simulink model "Galvo_sys_v13"  (R2013a)
settings: Solver=ode45  StartTime=0.0  StopTime=50e-3  MaxStep=1e-4  RelTol=1e-3
InitFcn:
  | Kp_cc = evalin('base','Kp_cc');
StartFcn:
  | Kp_cc = evalin('base','Kp_cc')
model workspace (MATLAB code in the model file):
  | Kp_cc = evalin('base','Kp_cc');
libraries: simulink x2
settings Model: Kp_cc=1  Creator=mainster  LastModifiedBy=mainster
settings DataIOCC: SaveFormat=StructureWithTime

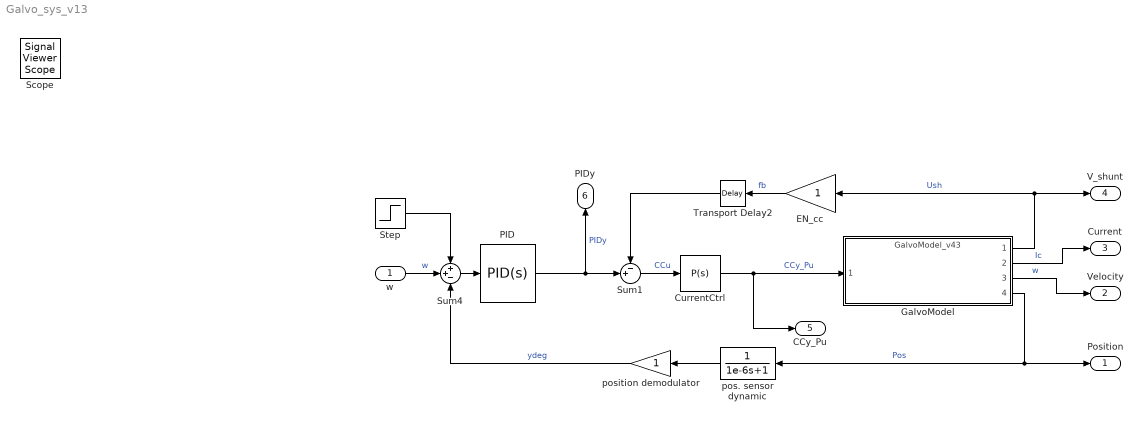
== system Galvo_sys_v13 ==
  w : Inport
  CurrentCtrl : simulink/Continuous/PID Controller  Controller=P  TimeDomain=Continuous-time  SampleTime=1  IntegratorMethod=Forward Euler  FilterMethod=Forward Euler  Form=Parallel  P=Kp_cc  I=1  D=0  N=100  InitialConditionSource=internal  InitialConditionForIntegrator=0  InitialConditionForFilter=0  ExternalReset=none  LimitOutput=on  UpperSaturationLimit=25  LowerSaturationLimit=-25  LinearizeAsGain=on  AntiWindupMode=none  Kb=1  TrackingMode=off  Kt=1  PParamMin=[]  PParamMax=[]  IParamMin=[]  IParamMax=[]  DParamMin=[]  DParamMax=[]  NParamMin=[]  NParamMax=[]  KbParamMin=[]  KbParamMax=[]  KtParamMin=[]  KtParamMax=[]  POutMin=[]  POutMax=[]  IOutMin=[]  IOutMax=[]  DOutMin=[]  DOutMax=[]  NOutMin=[]  NOutMax=[]  KbOutMin=[]  KbOutMax=[]  KtOutMin=[]  KtOutMax=[]  IntegratorOutMin=[]  IntegratorOutMax=[]  FilterOutMin=[]  FilterOutMax=[]  SumOutMin=[]  SumOutMax=[]  SumI1OutMin=[]  SumI1OutMax=[]  SumI2OutMin=[]  SumI2OutMax=[]  SumI3OutMin=[]  SumI3OutMax=[]  SumDOutMin=[]  SumDOutMax=[]  SaturationOutMin=[]  SaturationOutMax=[]  IntegratorContinuousStateAttributes=''  IntegratorStateMustResolveToSignalObject=off  IntegratorRTWStateStorageClass=Auto  FilterContinuousStateAttributes=''  FilterStateMustResolveToSignalObject=off  FilterRTWStateStorageClass=Auto
      settings: AttributesFormatString=Kp_cc = %<P>\nUccLim = +-%<UpperSaturationLimit>
  EN_cc : Gain
  GalvoModel : ModelReference  ModelNameDialog=GalvoModel_v43.slx  SimulationMode=Normal  Variant=on  OverrideUsingVariant=GalvoModel_v43  ModelReferenceVersion=1.40  CopyOfModelName=GalvoModel_v43.slx  DefaultDataLogging=on
      mask Display:
      | str=sprintf('%s',get(gcbh,'ModelName'));
      | port_label('input', 1, 'VCoil','texmode','on')
      | color('blue');
      | port_label('output', 1, 'VShunt','texmode','on')
      | color('black');
      | port_label('output', 2, 'Current')
      | port_label('output', 3, 'Velocity')
      | port_label('output', 4, 'Position')
      | %text(.05,.98,['{\fontsize{12}\it\bf' strrep(str,'_',' ') '}'],'horizontalAlignment','left','verticalAlignment','top','texmode','on')
      | text(.015,.98,['{\fontsize{12}\it\bf' strrep(str,'_','\_') '}'],'horizontalAlignment','left','verticalAlignment','top','texmode','on')
  PID : simulink/Continuous/PID Controller  Controller=PID  TimeDomain=Continuous-time  SampleTime=1  IntegratorMethod=Forward Euler  FilterMethod=Forward Euler  Form=Ideal  P=22.5419416589764  I=17.1686922499922  D=0.000772308769270681  N=7253.10376400166  InitialConditionSource=internal  InitialConditionForIntegrator=0  InitialConditionForFilter=0  ExternalReset=none  IgnoreLimit=on  LimitOutput=on  UpperSaturationLimit=2.5  LowerSaturationLimit=-2.5  LinearizeAsGain=on  AntiWindupMode=back-calculation  Kb=6  TrackingMode=off  Kt=0  PParamMin=[]  PParamMax=[]  IParamMin=[]  IParamMax=[]  DParamMin=[]  DParamMax=[]  NParamMin=[]  NParamMax=[]  KbParamMin=[]  KbParamMax=[]  KtParamMin=[]  KtParamMax=[]  POutMin=[]  POutMax=[]  IOutMin=[]  IOutMax=[]  DOutMin=[]  DOutMax=[]  NOutMin=[]  NOutMax=[]  KbOutMin=[]  KbOutMax=[]  KtOutMin=[]  KtOutMax=[]  IntegratorOutMin=[]  IntegratorOutMax=[]  FilterOutMin=[]  FilterOutMax=[]  SumOutMin=[]  SumOutMax=[]  SumI1OutMin=[]  SumI1OutMax=[]  SumI2OutMin=[]  SumI2OutMax=[]  SumI3OutMin=[]  SumI3OutMax=[]  SumDOutMin=[]  SumDOutMax=[]  SaturationOutMin=[]  SaturationOutMax=[]  IntegratorContinuousStateAttributes=''  IntegratorStateMustResolveToSignalObject=off  IntegratorRTWStateStorageClass=Auto  FilterContinuousStateAttributes=''  FilterStateMustResolveToSignalObject=off  FilterRTWStateStorageClass=Auto
      settings: AttributesFormatString=AWM=%<AntiWindupMode>\nD=%<D>\nI=%<I>\nN=%<N>\nP=%<P>\nLimit=+-%<UpperSaturationLimit>
  Step : Step  Time=1e-3  SampleTime=0  ZeroCross=off
      settings: AttributesFormatString=Ampl.: %<After>
  Sum1 : Sum  Inputs=-+|
  Sum4 : Sum  Inputs=++-
  Transport Delay2 : TransportDelay  DelayTime=1e-9
      settings: AttributesFormatString=Delay=%<DelayTime>
  pos. sensor dynamic : TransferFcn  Denominator=[1e-6 1]
  position demodulator : Gain
  Position : Outport
  Velocity : Outport  Port=2
  Current : Outport  Port=3
  V_shunt : Outport  Port=4
  CCy_Pu : Outport  Port=5
  PIDy : Outport  Port=6
  Scope : SignalViewerScope  IOType=viewer  NumInputPorts=4  LegendLocations=|  RefreshTime=0.035000
      | 0.78514      0.9169     0.17171    0.028289
      | 0.80649     0.68494     0.15036    0.028289
      |       0           0           0           0
      |       0           0           0           0
      settings: ShowLegends=on  YMin=-5~-5~-5~-5  YMax=5~5~5~5
  wires:
  Sum4/1 -> PID/1
  Step/1 -> Sum4/1
  w/1 -> Sum4/2  "w"
  position demodulator/1 -> Sum4/3  "ydeg"
  GalvoModel/1 -> V_shunt/1, EN_cc/1  "Ush"
  Sum1/1 -> CurrentCtrl/1  "CCu"
  PID/1 -> Sum1/2, PIDy/1  "PIDy"
  EN_cc/1 -> Transport Delay2/1  "fb"
  CurrentCtrl/1 -> GalvoModel/1, CCy_Pu/1  "CCy_Pu"
  Transport Delay2/1 -> Sum1/1
  pos. sensor dynamic/1 -> position demodulator/1
  GalvoModel/4 -> Position/1, pos. sensor dynamic/1  "Pos"
  GalvoModel/2 -> Current/1  "Ic"
  GalvoModel/3 -> Velocity/1  "w"
